simulink model "CSTR"  (Simulink 8.5)
settings: Solver=ode45  StartTime=0.0  StopTime=2  RelTol=1e-3
undefined symbols (not defined in the file): alpha, delta, u0, u_max, u_min
settings Model: Creator=ironi  LastModifiedBy=ironi
settings DataIOCC: SignalLoggingSaveFormat=Dataset
settings OptimizationCC: ExpressionDepthLimit=128
settings DebuggingCC: UnderspecifiedInitializationDetection=Simplified  MergeDetectMultiDrivingBlocksExec=error  FcnCallInpInsideContextMsg=EnableAllAsError  StateNameClashWarn=none
settings GRTTargetCC: CombineOutputUpdateFcns=on  GRTInterface=off

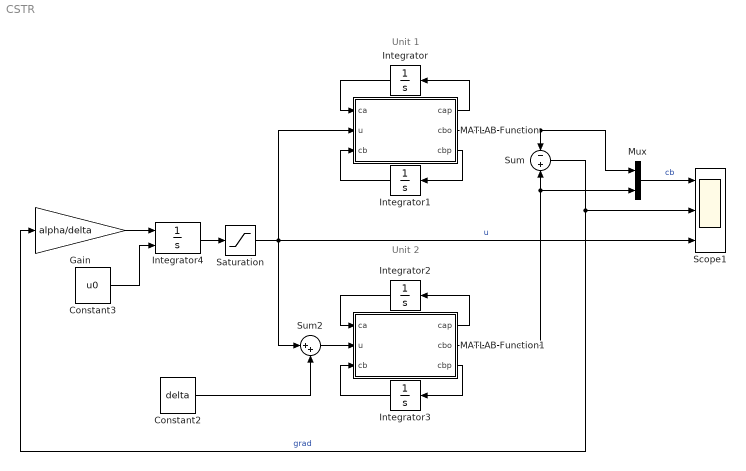
== system CSTR ==
  note: Unit 1
  note: Unit 2
  Constant2 : Constant  Value=delta
  Constant3 : Constant  Value=u0
  Gain : Gain  Gain=alpha/delta
  Integrator{,1..3} (4 alike) : Integrator
  Integrator4 : Integrator  InitialConditionSource=external  InitialCondition=15
  MATLAB Function : MATLAB Function  TreatAsAtomicUnit=on
  MATLAB Function1 : MATLAB Function  TreatAsAtomicUnit=on
  Mux : Mux  Inputs=2
  Saturation : Saturate  UpperLimit=u_max  LowerLimit=u_min
  Scope1 : Scope  NumInputPorts=3
      settings: YMin=-5~-5~-5  YMax=5~5~5  SaveName=sim_multi
  Sum : Sum  Inputs=-|+
  Sum2 : Sum  Inputs=|++
  wires:
  MATLAB Function/1(cap) -> Integrator/1
  MATLAB Function/3(cbp) -> Integrator1/1
  Integrator/1 -> MATLAB Function/1(ca)
  Integrator1/1 -> MATLAB Function/3(cb)
  MATLAB Function1/1(cap) -> Integrator2/1
  MATLAB Function1/3(cbp) -> Integrator3/1
  Integrator2/1 -> MATLAB Function1/1(ca)
  Integrator3/1 -> MATLAB Function1/3(cb)
  MATLAB Function/2(cbo) -> Sum/1, Mux/1
  MATLAB Function1/2(cbo) -> Sum/2, Mux/2
  Sum2/1 -> MATLAB Function1/2(u)
  Sum/1 -> Gain/1, Scope1/2  "grad"
  Gain/1 -> Integrator4/1
  Constant3/1 -> Integrator4/2
  Integrator4/1 -> Saturation/1
  Saturation/1 -> MATLAB Function/2(u), Sum2/1, Scope1/3  "u"
  Mux/1 -> Scope1/1  "cb"
  Constant2/1 -> Sum2/2

== matlab function MATLAB Function1 ==
  data: ca input double; u input double; cb input double; cap output double; cbo output double; cbp output double
function [cap, cbo, cbp]= fcn(ca, u, cb)
k1 = 24;
k2 = 24;
k3 = .5;
ca_in = 1;
cap = -k1*ca - 2*k3*ca^2 + u*(ca_in - ca);
cbp = k1*ca -k2*cb -u*cb;
cbo = cb;

== matlab function MATLAB Function ==
  data: ca input double; u input double; cb input double; cap output double; cbo output double; cbp output double
function [cap, cbo, cbp]= fcn(ca, u, cb)
k1 = 24;
k2 = 24;
k3 = .5;
ca_in = 1;
cap = -k1*ca - 2*k3*ca^2 + u*(ca_in - ca);
cbp = k1*ca -k2*cb -u*cb;
cbo = cb;
